simulink model "gen_rec"  (R2014a)
settings: Solver=ode23t  StartTime=2.7  StopTime=3.2  RelTol=1e-6
settings Model: Creator=Maryam  LastModifiedBy=mary

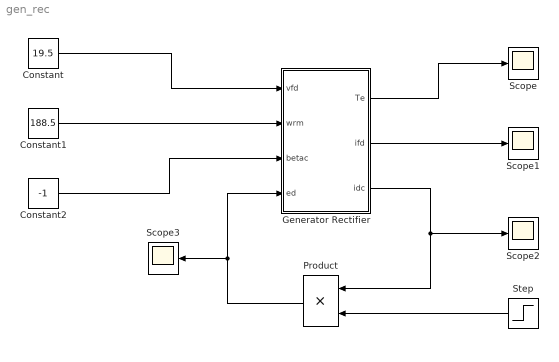
== system gen_rec ==
  Constant : Constant  Value=19.5
  Constant1 : Constant  Value=188.5
  Constant2 : Constant  Value=-1
  Generator Rectifier : Subsystem
  Product : Product
  Scope{,1..3} (4 alike) : Scope
      Scope settings: TimeRange=0.5  YMin=-0.3  YMax=1.3  MaxDataPoints=1000000
      Scope1 settings: YMin=174  YMax=187  MaxDataPoints=1000000
      Scope2 settings: YMin=0.000235123  YMax=0.000235135  SaveName=ScopeData2  MaxDataPoints=1000000
      Scope3 settings: SaveName=ScopeData3  MaxDataPoints=1000000
  Step : Step  Time=2.8  Before=21  After=3.39  SampleTime=0
  wires:
  Constant/1 -> Generator Rectifier/1(vfd)
  Constant1/1 -> Generator Rectifier/2("wrm ")
  Constant2/1 -> Generator Rectifier/3(betac)
  Product/1 -> Scope3/1, Generator Rectifier/4(ed)
  Generator Rectifier/1(Te) -> Scope/1
  Generator Rectifier/2(ifd) -> Scope1/1
  Generator Rectifier/3(idc) -> Product/1, Scope2/1
  Step/1 -> Product/2

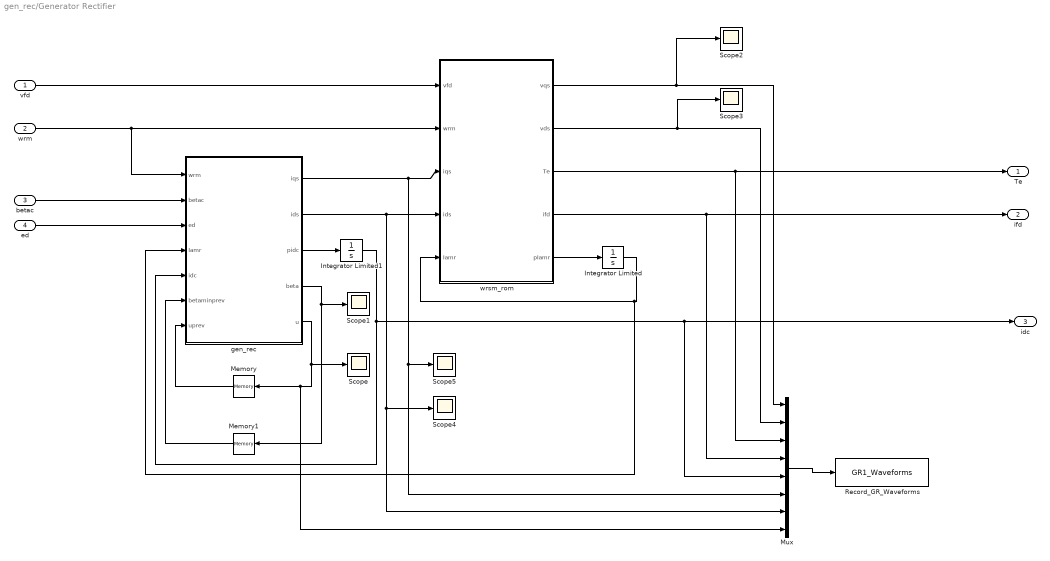
== system gen_rec/Generator Rectifier ==
  vfd : Inport
  "wrm " : Inport  Port=2
  betac : Inport  Port=3
  ed : Inport  Port=4
  Integrator Limited : Integrator  LimitOutput=on  UpperSaturationLimit=1  LowerSaturationLimit=0
  Integrator Limited1 : Integrator  LimitOutput=on  UpperSaturationLimit=1  LowerSaturationLimit=0
  Memory : Memory
  Memory1 : Memory
  Mux : Mux  Inputs=8
  Record_GR_Waveforms : ToWorkspace  VariableName=GR1_Waveforms  SaveFormat=Timeseries  SampleTime=-1
  Scope{,1..5} (6 alike) : Scope
      Scope settings: SaveName=ScopeData4
      Scope1 settings: SaveName=ScopeData5
      Scope2 settings: TimeRange=0.00277852449201843  YMin=-243.6253250957919  YMax=-242.9327837496225  SaveName=ScopeData6
      Scope3 settings: SaveName=ScopeData7
      Scope4 settings: SaveName=ScopeData8
      Scope5 settings: YMin=-14  YMax=0  SaveName=ScopeData9
  gen_rec : MATLAB Function  TreatAsAtomicUnit=on
  wrsm_rom : MATLAB Function  TreatAsAtomicUnit=on
  Te : Outport
  ifd : Outport  Port=2
  idc : Outport  Port=3
  wires:
  gen_rec/5(u) -> Scope/1, Mux/8, Memory/1
  Integrator Limited/1 -> gen_rec/4(Iamr), wrsm_rom/5(Iamr)
  vfd/1 -> wrsm_rom/1(vfd)
  wrsm_rom/5(pIamr) -> Integrator Limited/1
  "wrm "/1 -> gen_rec/1(wrm), wrsm_rom/2(wrm)
  gen_rec/2(ids) -> Scope4/1, Mux/7, wrsm_rom/4(ids)
  Memory/1 -> gen_rec/7(uprev)
  wrsm_rom/1(vqs) -> Scope2/1, Mux/1
  Memory1/1 -> gen_rec/6(betaminprev)
  gen_rec/1(iqs) -> Scope5/1, Mux/6, wrsm_rom/3(iqs)
  gen_rec/3(pidc) -> Integrator Limited1/1
  Integrator Limited1/1 -> idc/1, Mux/5, gen_rec/5(idc)
  betac/1 -> gen_rec/2(betac)
  wrsm_rom/2(vds) -> Scope3/1, Mux/2
  wrsm_rom/3(Te) -> Te/1, Mux/3
  Mux/1 -> Record_GR_Waveforms/1
  wrsm_rom/4(ifd) -> ifd/1, Mux/4
  ed/1 -> gen_rec/3(ed)
  gen_rec/4(beta) -> Scope1/1, Memory1/1

== matlab function gen_rec/Generator Rectifier/gen_rec ==
  data: iqs output; wrm input; betac input; ed input; Iamr input size=7; idc input; betaminprev input; uprev input; ids output; pidc output; beta output; u output; P parameter
function [iqs, ids, pidc, beta, u] = gen_rec(wrm, betac, ed, Iamr, idc, betaminprev, uprev,P)
%This routine represents the synchronous machine load-commutated rectifier.

%Inputs:
%wrm                            = Mechanical rotor speed (rad/sec)
%betac                          = Desired value of the firing angle (rad)
%ed                             = Output voltage (V)
%lmar                           = state vector for the flux linkages
%lamr(1)                        = Q-axis flux linkage
%lamr(2)                        = Q-axis flux linkage
%lamr(3)                        = Q-axis flux linkage
%lamr(4)                        = D-axis flux linkage
%lamr(5)                        = D-axis flux linkage
%lamr(6)                        = D-axis flux linkage
%lamr(7)                        = field flux linkage
%idc                            = dc link current (A)
%betaminprev                    = minimum firing angle in the previous
%                                 iteration
%uprev                          = commutation angle in the previous
%                                 iteration

%Outputs:
%iqs                            = Q-axis current (A)
%ids                            = D-axis current (A)
%pidc                           = time derivative of the dc link current
%beta                           = firing angle (rad)
%u                              = commutation angle (rad)

%Internal:
%wr                             = electrical rotor speed (rad/sec)

% Written by Maryam Alibeik
% Department of Electrical and Computer Engineering
% Purdue School of Engineering and Technology, IUPUI
% 723 West Michigan St. SL 113
% Indianapolis, IN 46202
% PH: 317-370-5153
% Email: malibeik@purdue.edu

%---------------------------------------------------------------------------

%Extracting the state vector
lamq1=Iamr(1);
lamq2=Iamr(2);
lamq3=Iamr(3);
lamd1=Iamr(4);
lamd2=Iamr(5);
lamd3=Iamr(6);
lamdf=Iamr(7);

%Calculation of the electrical rotor speed (radian/sec)
wr=(P.pole/2)*wrm;


%Calculation of the subtransient inductances
LdDP=P.Lls+1/((1/P.Lmd)+(1/P.Llfd)+sum(1./[P.Lld1;P.Lld2;P.Lld3]));
LqDP=P.Lls+1/((1/P.Lmq)+sum(1./[P.Lld1;P.Lld2;P.Lld3]));

%Calculation of the subtransient flux linkages
lamdDP=(LdDP-P.Lls)*((lamdf/P.Llfd)+sum([lamd1;lamd2;lamd3]./[P.Lld1;P.Lld2;P.Lld3]));
lamqDP=(LqDP-P.Lls)*sum([lamq1;lamq2;lamq3]./[P.Llq1;P.Llq2;P.Llq3]);

%Finding beta (Using Newton-Raphson Method) <-- Begin
% setup parameters for Newton Method
x = betaminprev; %initial value
epsilon = 1e-5;
delta = 1e-10;
max_iter = 100;
record = zeros(1,max_iter);

fx = sqrt(3)*lamqDP*cos(x)+sqrt(3)*lamdDP*sin(x)+2*idc*(LqDP-LdDP)*sin(2*x-pi/3);

for n=1:max_iter
    
    fp = -sqrt(3)*lamqDP*sin(x)+sqrt(3)*lamdDP*cos(x)+4*idc*(LqDP-LdDP)*cos(2*x-pi/3);
    if fp<delta
        disp('derivative too small (Newton Method - Beta)')
        break;
    end
    
    d = fx/fp;
    x = x - d;
    
    fx = sqrt(3)*lamqDP*cos(x)+sqrt(3)*lamdDP*sin(x)+2*idc*(LqDP-LdDP)*sin(2*x-pi/3);
    if abs(d)<epsilon
        
        break;
    end
    record(n) = x;
    
end
% betaminprev=x;
% betamin=betaminprev;
betamin=x;
beta=betamin;


%%Finding beta (Using Newton-Raphson Method) <-- End


eqDP=wr*lamdDP;
edDP=-wr*lamqDP;
phi=angle(eqDP-1i*edDP);
alpha=beta+phi;
Epk=sqrt((eqDP)^2+(edDP)^2);
Lc=(1/2)*(LqDP+LdDP)+(LdDP-LqDP)*sin(2*beta+pi/6);
Lt=LqDP+LdDP+(LdDP-LqDP)*sin(2*beta-pi/6);
K=sqrt(3)*(-lamqDP*sin(beta)+lamqDP*cos(beta))+((LdDP-LqDP)*cos(2*beta+2*pi/3)-0.5*(LqDP+LdDP))*idc;


%Finding U --< Newton Begin
% setup parameters for Newton Method
x = uprev; %initial value
epsilon = 1e-5;
delta = 1e-10;
max_iter = 100;
record = zeros(1,max_iter);

fx = K-sqrt(3)*(-lamqDP*sin(beta+x)+lamdDP*cos(beta+x))-((LqDP-LdDP)*sin(2*beta+2*x-2*pi/3)+0.5*(LqDP+LdDP))*idc;

for n=1:max_iter
    
    fp = sqrt(3)*lamqDP*cos(beta+x)+sqrt(3)*lamdDP*sin(beta+x)-(2*(LqDP-LdDP)*cos(2*beta+2*x-2*pi/3))*idc;
    if fp<delta
        disp('derivative too small (Newton Method - U)')
        break;
    end
    
    d = fx/fp;
    x = x - d;
    
    fx = K-sqrt(3)*(-lamqDP*sin(beta+x)+lamdDP*cos(beta+x))-((LqDP-LdDP)*sin(2*beta+2*x-2*pi/3)+0.5*(LqDP+LdDP))*idc;
    if abs(d)<epsilon
 
        break;
    end
    record(n) = x;
    
end
%uprev=x;
u=x;

%Finding U --< Newton End

%calculation of q and d axis current during conduction
iqsCond=(2*sqrt(3)/pi)*idc*(cos(beta+2*pi/3)-cos(beta+u+(pi/3)));
idsCond=(2*sqrt(3)/pi)*idc*(sin(beta+2*pi/3)-sin(beta+u+(pi/3)));

%thetar=0
theta=0;
ias1=((K+sqrt(3)*(lamqDP*sin(theta+beta)-lamdDP*cos(theta+beta))/((LqDP+LdDP)-(LqDP-LdDP)*cos(2*theta+2*beta)))-(((LqDP-LdDP)*cos(2*theta+2*beta-2*pi/3)+0.5*(LqDP+LdDP))*idc/((LqDP+LdDP)-(LqDP-LdDP)*cos(2*theta+2*beta))));
iqs1=(2*sqrt(3)/3)*(-ias1*sin(theta+beta)-idc*sin(theta+beta+pi/3));
ids1=(2*sqrt(3)/3)*(ias1*cos(theta+beta)+idc*cos(theta+beta+pi/3));
%thetar=u/4
theta=u/4;
ias2=((K+sqrt(3)*(lamqDP*sin(theta+beta)-lamdDP*cos(theta+beta))/((LqDP+LdDP)-(LqDP-LdDP)*cos(2*theta+2*beta)))-(((LqDP-LdDP)*cos(2*theta+2*beta-2*pi/3)+0.5*(LqDP+LdDP))*idc/((LqDP+LdDP)-(LqDP-LdDP)*cos(2*theta+2*beta))));
iqs2=(2*sqrt(3)/3)*(-ias2*sin(theta+beta)-idc*sin(theta+beta+pi/3));
ids2=(2*sqrt(3)/3)*(ias2*cos(theta+beta)+idc*cos(theta+beta+pi/3));
%thetar=u/2
theta=u/2;
ias3=((K+sqrt(3)*(lamqDP*sin(theta+beta)-lamdDP*cos(theta+beta))/((LqDP+LdDP)-(LqDP-LdDP)*cos(2*theta+2*beta)))-(((LqDP-LdDP)*cos(2*theta+2*beta-2*pi/3)+0.5*(LqDP+LdDP))*idc/((LqDP+LdDP)-(LqDP-LdDP)*cos(2*theta+2*beta))));
iqs3=(2*sqrt(3)/3)*(-ias3*sin(theta+beta)-idc*sin(theta+beta+pi/3));
ids3=(2*sqrt(3)/3)*(ias3*cos(theta+beta)+idc*cos(theta+beta+pi/3));
%thetar=3*u/4
theta=3*u/4;
ias4=((K+sqrt(3)*(lamqDP*sin(theta+beta)-lamdDP*cos(theta+beta))/((LqDP+LdDP)-(LqDP-LdDP)*cos(2*theta+2*beta)))-(((LqDP-LdDP)*cos(2*theta+2*beta-2*pi/3)+0.5*(LqDP+LdDP))*idc/((LqDP+LdDP)-(LqDP-LdDP)*cos(2*theta+2*beta))));
iqs4=(2*sqrt(3)/3)*(-ias4*sin(theta+beta)-idc*sin(theta+beta+pi/3));
ids4=(2*sqrt(3)/3)*(ias4*cos(theta+beta)+idc*cos(theta+beta+pi/3));
%thetar=u
theta=u;
ias5=((K+sqrt(3)*(lamqDP*sin(theta+beta)-lamdDP*cos(theta+beta))/((LqDP+LdDP)-(LqDP-LdDP)*cos(2*theta+2*beta)))-(((LqDP-LdDP)*cos(2*theta+2*beta-2*pi/3)+0.5*(LqDP+LdDP))*idc/((LqDP+LdDP)-(LqDP-LdDP)*cos(2*theta+2*beta))));
iqs5=(2*sqrt(3)/3)*(-ias5*sin(theta+beta)-idc*sin(theta+beta+pi/3));
ids5=(2*sqrt(3)/3)*(ias5*cos(theta+beta)+idc*cos(theta+beta+pi/3));


iqs_C=[iqs1 iqs2 iqs3 iqs4 iqs5]';
ids_C=[ids1 ids2 ids3 ids4 ids5]';
iqsCommu=(u/4*pi)*(iqs_C(1)+4*iqs_C(2)+2*iqs_C(3)+4*iqs_C(4)+iqs_C(5));
idsCommu=(u/4*pi)*(ids_C(1)+4*ids_C(2)+2*ids_C(3)+4*ids_C(4)+ids_C(5));

iqs=iqsCond+iqsCommu;
ids=idsCond+idsCommu;


pidc=((3*sqrt(3)/pi)*Epk*cos(alpha)-ed-(P.rl+(3/pi)*wr*Lc)*idc)/(P.Ll+Lt);

end

== matlab function gen_rec/Generator Rectifier/wrsm_rom ==
  data: vfd input; vqs output; wrm input; iqs input; ids input; Iamr input size=7; vds output; Te output; ifd output; pIamr output size=7; P parameter
function [vqs, vds, Te, ifd, pIamr] = wrsm_rom(vfd, wrm, iqs, ids, Iamr,P)
%This routine represents reduce order model of the synchronous load fed
%commutated rectifier.

%Inputs:
%vfd                            = field voltage (V)
%wrm                            = mechanical rotor speed (rad/sec)
%iqs                            = Q-axis current (A)
%ids                            = D-axis current (A) 
%lmar                           = state vector for the flux linkages
%lamr(1)                        = Q-axis flux linkage
%lamr(2)                        = Q-axis flux linkage
%lamr(3)                        = Q-axis flux linkage
%lamr(4)                        = D-axis flux linkage
%lamr(5)                        = D-axis flux linkage
%lamr(6)                        = D-axis flux linkage
%lamr(7)                        = field flux linkage

%Outputs:
%vqs                            = Q-axis voltage (V)
%vds                            = D-axis voltage (V)
%Te                             = Electrical torque
%ifd                            = field current (A)
%pIamr                          = Time derivative of the state vectors
%plamr(1)                        = Time derivative of Q-axis flux linkage
%plamr(2)                        = Time derivative of Q-axis flux linkage
%plamr(3)                        = Time derivative of Q-axis flux linkage
%plamr(4)                        = Time derivative of D-axis flux linkage
%plamr(5)                        = Time derivative of D-axis flux linkage
%plamr(6)                        = Time derivative of D-axis flux linkage
%plamr(7)                        = Time derivative of field flux linkage

%Internal:
%wr                             = electrical rotor speed (rad/sec)

% Written by Maryam Alibeik
% Department of Electrical and Computer Engineering
% Purdue School of Engineering and Technology, IUPUI
% 723 West Michigan St. SL 113
% Indianapolis, IN 46202
% PH: 317-370-5153
% Email: malibeik@purdue.edu

lamq1=Iamr(1);
lamq2=Iamr(2);
lamq3=Iamr(3);
lamd1=Iamr(4);
lamd2=Iamr(5);
lamd3=Iamr(6);
lamdf=Iamr(7);

%calculation of the magnetizing Q and D axis currents
imq=(iqs+sum([lamq1,lamq2,lamq3]./[P.Llq1,P.Llq2,P.Llq3]))/(1+P.Lmq*sum(1./[P.Llq1,P.Llq2,P.Llq3]));
imd=(ids+(lamdf/P.Llfd)+sum([lamd1,lamd2,lamd3]./[P.Lld1,P.Lld2,P.Lld3]))/(1+P.Lmd*((1/P.Llfd)+sum(1./[P.Lld1,P.Lld2,P.Lld3])));
iq1=(lamq1-P.Lmq*imq)/P.Llq1;
iq2=(lamq2-P.Lmq*imq)/P.Llq2;
iq3=(lamq3-P.Lmq*imq)/P.Llq3;
id1=(lamd1-P.Lmd*imd)/P.Lld1;
id2=(lamd2-P.Lmd*imd)/P.Lld2;
id3=(lamd3-P.Lmd*imd)/P.Lld3;
ifd=(lamdf-P.Lmd*imd)/P.Llfd;

%Calculation of the q axis rotor flux linkages
plamq1=-P.rq1*iq1;
plamq2=-P.rq2*iq2;
plamq3=-P.rq3*iq3;

%Calculation of the d axis rotor flux linkages
plamd1=-P.rd1*id1;
plamd2=-P.rd2*id2;
plamd3=-P.rd3*id3;

%Calculation of the field flux linkages
plamdf=vfd-P.rfd*ifd;

%Pack the time derivatives of the state vectors
pIamr=[plamq1,plamq2,plamq3,plamd1,plamd2,plamd3,plamdf]';

%calculation of the magnetizing q and d axis flux linkages
lamMq=P.Lmq*imq;
lamMd=P.Lmd*imd;

%Calculation of the electrical rotor speed (radian/sec)
wr=(P.pole/2)*wrm;

%Calculation of the electrical rotor speed (degree/sec)
Te=1.5*(P.pole/2)*(lamMd*imq-lamMq*imd);

lamqS=P.Lls*iqs+P.Lmq*imq;
lamdS=P.Lls*ids+P.Lmd*imd;
vqs=P.rs*iqs+wr*lamdS;
vds=P.rs*ids-wr*lamqS;
